simulink model "Sposob_3a"  (R2022b)
settings: Solver=ode4  StartTime=0.0  StopTime=10.0  FixedStep=0.1  RelTol=1e-3
values from neighbouring files (symbols this model uses):
  k = 6    [Sposob1.mat]    (also in Sposob2a.mat; Sposob2b.mat; Sposob3a.mat; Sposob3b.mat)
  m = 14    [Sposob1.mat]    (also in Sposob2a.mat; Sposob2b.mat; Sposob3a.mat; Sposob3b.mat)
  x0 = 0.1    [Sposob1.mat]    (also in Sposob2a.mat = [0.1 0]; Sposob2b.mat = [0.1 0]; Sposob3a.mat = [0.1 0]; Sposob3b.mat = [0.1 0])
settings Model: Creator=student  LastModifiedBy=Jakub
settings DebuggingCC: UnconnectedInputMsg=warning  UnconnectedOutputMsg=warning  UnconnectedLineMsg=warning
settings ModelReferenceCC: EnableRefExpFcnMdlSchedulingChecks=on
settings RTWCC: DLArmComputeVersion=19.05

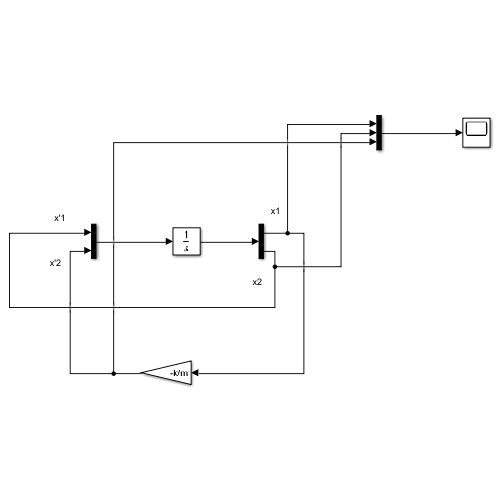
[thumbnail: Simulink's stored preview of the top-level diagram]
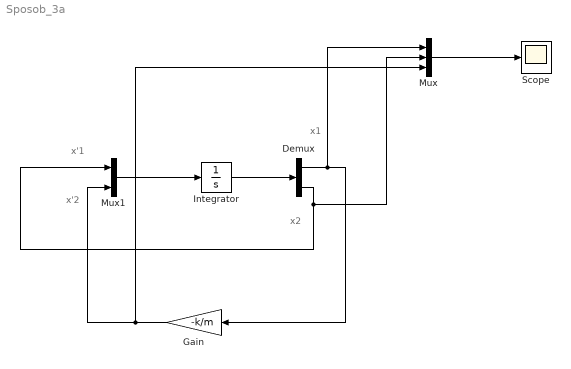
== system Sposob_3a ==
  note: x2
  note: x1
  note: x'2
  note: x'1
  Demux : Demux  Outputs=2
  Gain : Gain  Gain=-k/m
  Integrator : Integrator  InitialCondition=x0
  Mux : Mux  Inputs=3
  Mux1 : Mux  Inputs=2
  Scope : Scope
  wires:
  Integrator/1 -> Demux/1
  Mux1/1 -> Integrator/1
  Demux/1 -> Mux/1, Gain/1
  Demux/2 -> Mux1/1, Mux/2
  Gain/1 -> Mux/3, Mux1/2
  Mux/1 -> Scope/1
